simulink model "SC_Lab3_Variant3"  (R2025b)
settings: Solver=ode45  StartTime=0.0  StopTime=1  RelTol=1e-3
(part 1 of 2)
settings Model: Creator=m  LastModifiedBy=m
settings DataIOCC: SaveFormat=StructureWithTime

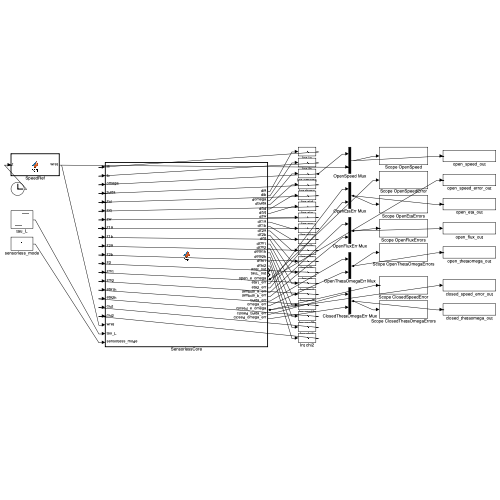
[thumbnail: Simulink's stored preview of the top-level diagram]
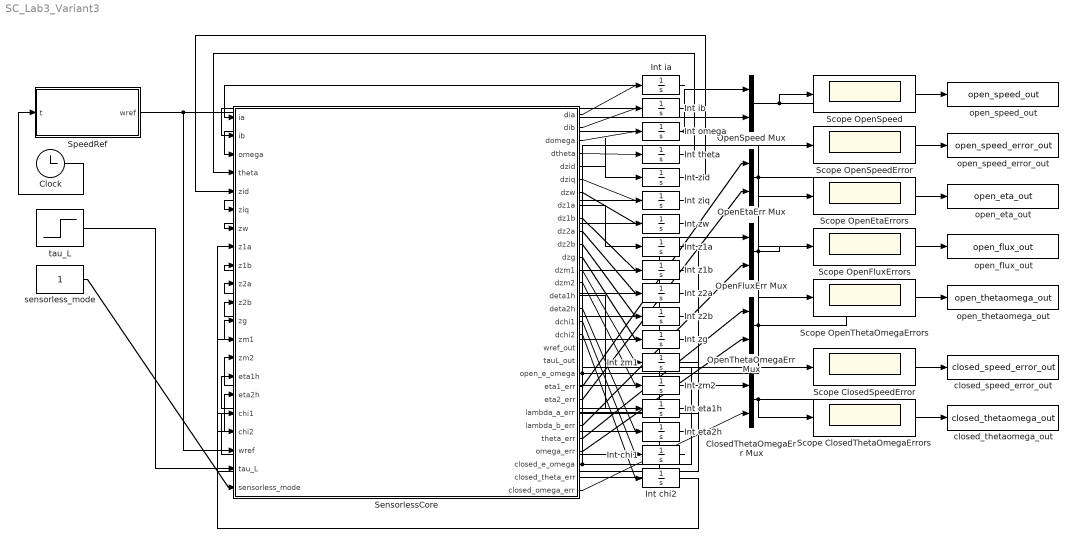
== system SC_Lab3_Variant3 ==
  Clock : Clock
  ClosedThetaOmegaErr Mux : Mux  Inputs=2
  Int chi1 : Integrator
  Int chi2 : Integrator
  Int eta1h : Integrator  InitialCondition=0.128
  Int eta2h : Integrator
  Int ia : Integrator
  Int ib : Integrator
  Int omega : Integrator
  Int theta : Integrator
  Int z1a : Integrator
  Int z1b : Integrator
  Int z2a : Integrator
  Int z2b : Integrator
  Int zg : Integrator
  Int zid : Integrator
  Int ziq : Integrator
  Int zm1 : Integrator
  Int zm2 : Integrator
  Int zw : Integrator
  OpenEtaErr Mux : Mux  Inputs=2
  OpenFluxErr Mux : Mux  Inputs=2
  OpenSpeed Mux : Mux  Inputs=2
  OpenThetaOmegaErr Mux : Mux  Inputs=2
  Scope ClosedSpeedError : Scope
  Scope ClosedThetaOmegaErrors : Scope
  Scope OpenEtaErrors : Scope
  Scope OpenFluxErrors : Scope
  Scope OpenSpeed : Scope
  Scope OpenSpeedError : Scope
  Scope OpenThetaOmegaErrors : Scope
  SensorlessCore : MATLAB Function  TreatAsAtomicUnit=on
  SpeedRef : MATLAB Function  TreatAsAtomicUnit=on
  closed_speed_error_out : ToWorkspace  VariableName=closed_speed_error_out  SaveFormat=Structure With Time  SampleTime=-1
  closed_thetaomega_out : ToWorkspace  VariableName=closed_thetaomega_out  SaveFormat=Structure With Time  SampleTime=-1
  open_eta_out : ToWorkspace  VariableName=open_eta_out  SaveFormat=Structure With Time  SampleTime=-1
  open_flux_out : ToWorkspace  VariableName=open_flux_out  SaveFormat=Structure With Time  SampleTime=-1
  open_speed_error_out : ToWorkspace  VariableName=open_speed_error_out  SaveFormat=Structure With Time  SampleTime=-1
  open_speed_out : ToWorkspace  VariableName=open_speed_out  SaveFormat=Structure With Time  SampleTime=-1
  open_thetaomega_out : ToWorkspace  VariableName=open_thetaomega_out  SaveFormat=Structure With Time  SampleTime=-1
  sensorless_mode : Constant
  tau_L : Step  Time=0.5  After=0.35  SampleTime=0
  wires:
  Clock/1 -> SpeedRef/1(t)
  SpeedRef/1(wref) -> SensorlessCore/19(wref), OpenSpeed Mux/2
  tau_L/1 -> SensorlessCore/20(tau_L)
  sensorless_mode/1 -> SensorlessCore/21(sensorless_mode)
  Int ia/1 -> SensorlessCore/1(ia)
  Int ib/1 -> SensorlessCore/2(ib)
  Int omega/1 -> SensorlessCore/3(omega), OpenSpeed Mux/1
  Int theta/1 -> SensorlessCore/4(theta)
  Int zid/1 -> SensorlessCore/5(zid)
  Int ziq/1 -> SensorlessCore/6(ziq)
  Int zw/1 -> SensorlessCore/7(zw)
  Int z1a/1 -> SensorlessCore/8(z1a)
  Int z1b/1 -> SensorlessCore/9(z1b)
  Int z2a/1 -> SensorlessCore/10(z2a)
  Int z2b/1 -> SensorlessCore/11(z2b)
  Int zg/1 -> SensorlessCore/12(zg)
  Int zm1/1 -> SensorlessCore/13(zm1)
  Int zm2/1 -> SensorlessCore/14(zm2)
  Int eta1h/1 -> SensorlessCore/15(eta1h)
  Int eta2h/1 -> SensorlessCore/16(eta2h)
  Int chi1/1 -> SensorlessCore/17(chi1)
  Int chi2/1 -> SensorlessCore/18(chi2)
  SensorlessCore/1(dia) -> Int ia/1
  SensorlessCore/2(dib) -> Int ib/1
  SensorlessCore/3(domega) -> Int omega/1
  SensorlessCore/4(dtheta) -> Int theta/1
  SensorlessCore/5(dzid) -> Int zid/1
  SensorlessCore/6(dziq) -> Int ziq/1
  SensorlessCore/7(dzw) -> Int zw/1
  SensorlessCore/8(dz1a) -> Int z1a/1
  SensorlessCore/9(dz1b) -> Int z1b/1
  SensorlessCore/10(dz2a) -> Int z2a/1
  SensorlessCore/11(dz2b) -> Int z2b/1
  SensorlessCore/12(dzg) -> Int zg/1
  SensorlessCore/13(dzm1) -> Int zm1/1
  SensorlessCore/14(dzm2) -> Int zm2/1
  SensorlessCore/15(deta1h) -> Int eta1h/1
  SensorlessCore/16(deta2h) -> Int eta2h/1
  SensorlessCore/17(dchi1) -> Int chi1/1
  SensorlessCore/18(dchi2) -> Int chi2/1
  OpenSpeed Mux/1 -> Scope OpenSpeed/1, open_speed_out/1
  SensorlessCore/21(open_e_omega) -> Scope OpenSpeedError/1, open_speed_error_out/1
  SensorlessCore/22(eta1_err) -> OpenEtaErr Mux/1
  SensorlessCore/23(eta2_err) -> OpenEtaErr Mux/2
  OpenEtaErr Mux/1 -> Scope OpenEtaErrors/1, open_eta_out/1
  SensorlessCore/24(lambda_a_err) -> OpenFluxErr Mux/1
  SensorlessCore/25(lambda_b_err) -> OpenFluxErr Mux/2
  OpenFluxErr Mux/1 -> Scope OpenFluxErrors/1, open_flux_out/1
  SensorlessCore/26(theta_err) -> OpenThetaOmegaErr Mux/1
  SensorlessCore/27(omega_err) -> OpenThetaOmegaErr Mux/2
  OpenThetaOmegaErr Mux/1 -> Scope OpenThetaOmegaErrors/1, open_thetaomega_out/1
  SensorlessCore/28(closed_e_omega) -> Scope ClosedSpeedError/1, closed_speed_error_out/1
  SensorlessCore/29(closed_theta_err) -> ClosedThetaOmegaErr Mux/1
  SensorlessCore/30(closed_omega_err) -> ClosedThetaOmegaErr Mux/2
  ClosedThetaOmegaErr Mux/1 -> Scope ClosedThetaOmegaErrors/1, closed_thetaomega_out/1

== matlab function SC_Lab3_Variant3/SpeedRef ==
  data: t input; wref output
function wref = fcn(t)
                     if t < 0.2            
                         wref = 530*t;     
                     else                  
                         wref = 106;       
                     end
